simulink model "data_read"  (R2025b)
settings: Solver=ode4  StartTime=0.0  StopTime=600  FixedStep=0.01  RelTol=1e-3
StartFcn:
  | % % StartFcn: ensure external udp reader is running and clear queue
  | % try
  | %     if ~evalin('base','exist(''udpportObj'',''var'')')
  | %         udp_reader_start; % starts udpport and configures callback
  | %     end
  | %     % clear queue to drop any leftover packets
  | %     if evalin('base','exist(''udpQueue'',''var'')')
  | %         q = evalin('base','udpQueue');
  | %         q.head = 1; q.tail = 1; q.count = 0;
  | %         assignin('base','udpQueue',q);
  | %     end
  | % catch ME
  | %     warning('StartFcn: failed to ensure UDP reader: %s', ME.message);
  | % end
model workspace (MAT data in the model file):
  data_prec = 1e-05
undefined symbols (not defined in the file): f
libraries: dspswit3 x5, simulink x1, sldrtlib x1, instrumentlib x1
settings Model: Creator=karol  LastModifiedBy=admin
settings SolverCC: ConcurrentTasks=on  PositivePriorityOrder=on  AutoInsertRateTranBlk=on
settings OptimizationCC: BlockReduction=off  OptimizeBlockIOStorage=off
settings DebuggingCC: TasksWithSamePriorityMsg=none
settings HardwareCC: ProdBitPerLong=64.0  ProdLongLongMode=on  ProdHWDeviceType=Intel->x86-64 (Linux 64)
settings RTWCC: SystemTargetFile=slrealtime.tlc  TemplateMakefile=slrealtime_default_tmf  Toolchain=Simulink Real-Time Toolchain  BuildConfiguration=Faster Runs  CodeExecutionProfiling=on  TargetLang=C++  GPUComputeCapability=3.5  Description=Simulink Real-Time
settings SimulinkRealTimeTargetCC: SLRTFileLogMaxRuns=1.0  ExtModeMaxTrigDuration=10.0  ExtModeStaticAllocSize=1000000.0  ExtModeTransport=0.0  MultiwordLength=2048.0  DynamicStringBufferSize=256.0  PreserveMATLABNamespacesInGeneratedCode=on  SubcomponentCodeInterfacePackaging=Reusable function  InstructionSetFMA=off  LogToMDFFile=off

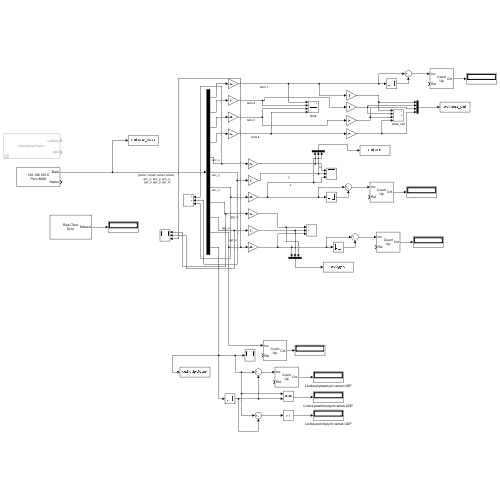
[thumbnail: Simulink's stored preview of the top-level diagram]
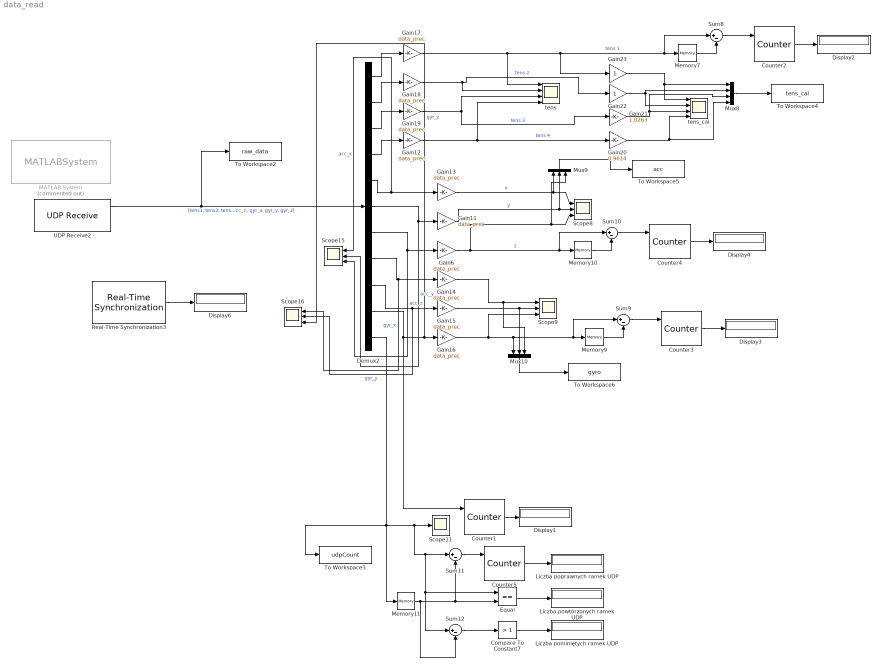
== system data_read ==
  Compare To Constant7 : simulink/Logic and Bit Operations/Compare To Constant  relop=>  const=1  OutDataTypeStr=boolean
  Counter1 : dspswit3/Counter  Direction=Up  CountEvent=Non-zero sample  CounterSize=User defined  MaxCount=100000  InitialCount=0  Output=Count  HitValue=32  ResetInput=on  SamplesPerFrame=1  Ts=1  CntDtype=int32  HitDtype=Logical
  Counter2 : dspswit3/Counter  Direction=Up  CountEvent=Non-zero sample  CounterSize=User defined  MaxCount=10000  InitialCount=0  Output=Count  HitValue=32  ResetInput=on  SamplesPerFrame=1  Ts=1  CntDtype=double  HitDtype=Logical
  Counter3 : dspswit3/Counter  Direction=Up  CountEvent=Non-zero sample  CounterSize=User defined  MaxCount=10000  InitialCount=0  Output=Count  HitValue=32  ResetInput=on  SamplesPerFrame=1  Ts=1  CntDtype=double  HitDtype=Logical
  Counter4 : dspswit3/Counter  Direction=Up  CountEvent=Non-zero sample  CounterSize=User defined  MaxCount=10000  InitialCount=0  Output=Count  HitValue=32  ResetInput=on  SamplesPerFrame=1  Ts=1  CntDtype=double  HitDtype=Logical
  Counter5 : dspswit3/Counter  Direction=Up  CountEvent=Non-zero sample  CounterSize=User defined  MaxCount=100000  InitialCount=0  Output=Count  HitValue=32  ResetInput=on  SamplesPerFrame=1  Ts=1  CntDtype=int32  HitDtype=Logical
  Demux2 : Demux  Outputs=11
  Display{1..4,6} (5 alike) : Display
  Equal : RelationalOperator  Operator===  OutDataTypeStr=boolean  RndMeth=Simplest  InputSameDT=off
  Gain{6,11,13..16} (6 alike) : Gain  Gain=data_prec  OutDataTypeStr=single
  Gain{12,17..19} (4 alike) : Gain  Gain=data_prec  OutDataTypeStr=double
  Gain20 : Gain  Gain=0.9614
  Gain21 : Gain  Gain=1.0263
  Gain22 : Gain
  Gain23 : Gain
  Liczba pominiętych ramek UDP : Display
  Liczba poprawnych ramek UDP : Display
  Liczba powtórzonych ramek UDP : Display
  MATLAB System : MATLABSystem  Commented=on  System=UdpQueueReader  Timeout=0  SimulateUsing=Interpreted execution
      mask Type: UdpQueueReader
  Memory{7,9..11} (4 alike) : Memory
  Mux10 : Mux  Inputs=3
  Mux8 : Mux
  Mux9 : Mux  Inputs=3
  Real-Time Synchronization3 : sldrtlib/Real-Time Synchronization  SampleTime=0.01  MaxMissedTicks=100000  ShowMissedTicks=on  YieldWhenWaiting=off
  Scope11 : Scope
      settings: ActiveDisplayYMinimum=24497.900073613906  ActiveDisplayYMaximum=24592.488868141339  DataLoggingVariableName=ScopeData12
  Scope{8..9,15..16} (4 alike) : Scope  NumInputPorts=3
      Scope15 settings: ActiveDisplayYMinimum=-127467.87499999997  ActiveDisplayYMaximum=1.120030875E+6  DataLoggingVariableName=ScopeData17
      Scope16 settings: ActiveDisplayYMinimum=-93853.625  ActiveDisplayYMaximum=35162.625  DataLoggingVariableName=ScopeData18
      Scope8 settings: ActiveDisplayYMinimum=-4.2882274091243744  ActiveDisplayYMaximum=11.889747232198715  DataLoggingVariableName=ScopeData9
      Scope9 settings: ActiveDisplayYMinimum=-119.15724563598633  ActiveDisplayYMaximum=80.090457916259766  DataLoggingVariableName=ScopeData10
  Sum{8..12} (5 alike) : Sum  Inputs=|+-
  To Workspace2 : ToWorkspace  VariableName=raw_data  SampleTime=-1
      settings: Save2DSignal=2-D array (concatenate along first dimension)
  To Workspace3 : ToWorkspace  VariableName=udpCount  SampleTime=-1
      settings: Save2DSignal=2-D array (concatenate along first dimension)
  To Workspace4 : ToWorkspace  VariableName=tens_cal  SampleTime=-1
      settings: Save2DSignal=2-D array (concatenate along first dimension)
  To Workspace5 : ToWorkspace  VariableName=acc  SampleTime=-1
      settings: Save2DSignal=2-D array (concatenate along first dimension)
  To Workspace6 : ToWorkspace  VariableName=gyro  SampleTime=-1
      settings: Save2DSignal=2-D array (concatenate along first dimension)
  UDP Receive2 : instrumentlib/UDP Receive  LocalAddress=192.168.100.5  LocalPort=8888  EnablePortSharing=on  Host=192.168.100.13  Port=8888  GetLatestData=off  DataSize=[ 1, 11 ]  DataType=int32  ASCIIFormatting=%f,  Terminator=LF  CustomTerminator=10  ByteOrder=little-endian  EnableBlockingMode=off  Timeout=10  SampleTime=0.01  SimulateUsing=Interpreted execution
  tens : Scope  NumInputPorts=4
      settings: ActiveDisplayYMinimum=-97.815363781047921  ActiveDisplayYMaximum=180.42207380726842
  tens_cal : Scope  NumInputPorts=4
      settings: ActiveDisplayYMinimum=-97.07907683856422  ActiveDisplayYMaximum=173.79549132491505  DataLoggingVariableName=ScopeData19
  wires:
  Demux2/4 -> Gain12/1
  Demux2/6 -> Scope15/2, Gain11/1  "acc_y"
  Demux2/1 -> Gain17/1
  Demux2/10 -> Counter1/1, Scope16/3, Gain16/1  "gyr_z"
  Demux2/7 -> Scope15/3, Gain6/1  "acc_z"
  Demux2/2 -> Gain18/1
  Demux2/3 -> Gain19/1
  Demux2/8 -> Scope16/1, Gain14/1  "gyr_x"
  Demux2/5 -> Gain13/1, Scope15/1  "acc_x"
  Demux2/9 -> Gain15/1, Scope16/2  "gyr_y"
  Gain17/1 -> tens/1, Gain23/1, Sum8/1, Memory7/1  "tens 1"
  Gain18/1 -> tens/2, Gain22/1  "tens 2"
  Gain19/1 -> tens/3, Gain21/1  "tens 3"
  Gain12/1 -> Gain20/1, tens/4  "tens 4"
  Gain13/1 -> Mux9/1, Scope8/1  "x"
  Gain11/1 -> Mux9/2, Scope8/2  "y"
  Gain6/1 -> Sum10/1, Memory10/1, Mux9/3, Scope8/3  "z"
  Gain14/1 -> Mux10/3, Scope9/1
  Gain15/1 -> Mux10/2, Scope9/2
  Gain16/1 -> Scope9/3, Mux10/1, Sum9/1, Memory9/1
  Counter1/1 -> Display1/1
  Memory7/1 -> Sum8/2
  Sum8/1 -> Counter2/1
  Counter2/1 -> Display2/1
  Memory9/1 -> Sum9/2
  Counter3/1 -> Display3/1
  Sum9/1 -> Counter3/1
  Counter4/1 -> Display4/1
  Memory10/1 -> Sum10/2
  Sum10/1 -> Counter4/1
  Demux2/11 -> To Workspace3/1, Memory11/1, Sum12/1, Equal/1, Sum11/1, Scope11/1
  Memory11/1 -> Sum12/2, Equal/2, Sum11/2
  Sum11/1 -> Counter5/1
  Counter5/1 -> Liczba poprawnych ramek UDP/1
  UDP Receive2/1 -> To Workspace2/1, Demux2/1  "[tens1, tens2, tens3, tens4,  acc_x, acc_y, acc_z,  gyr_x, gyr_y, gyr_z]"
  Gain23/1 -> Mux8/1, tens_cal/1
  Gain22/1 -> tens_cal/2, Mux8/2
  Gain21/1 -> Mux8/3, tens_cal/3
  Gain20/1 -> tens_cal/4, Mux8/4
  Mux8/1 -> To Workspace4/1
  Mux9/1 -> To Workspace5/1
  Mux10/1 -> To Workspace6/1
  Real-Time Synchronization3/1 -> Display6/1
  Equal/1 -> Liczba powtórzonych ramek UDP/1
  Sum12/1 -> Compare To Constant7/1
  Compare To Constant7/1 -> Liczba pominiętych ramek UDP/1
